simulink model "hearing_aid_final_model"  (R2018b)
settings: Solver=VariableStepAuto  StartTime=0.0  StopTime=67  RelTol=1e-3
libraries: dspvision x2, simulink x1, dspsnks4 x1, dspadpt3 x1
settings Model: Creator=User  LastModifiedBy=User

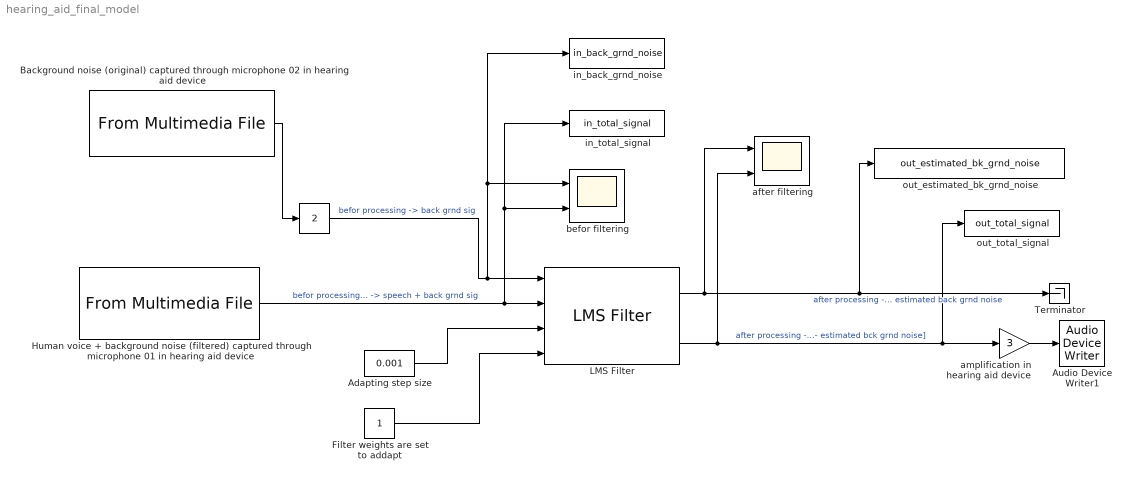
== system hearing_aid_final_model ==
  " " : simulink/Math Operations/Slider Gain  gain=2  low=0  high=5
  Adapting step size : Constant  Value=0.001  OutDataTypeStr=Inherit: Inherit via back propagation
  Audio Device Writer1 : dspsnks4/Audio Device Writer  Driver=DirectSound  Device=Default  InheritSampleRate=on  SampleRate=44100  BitDepth=16-bit integer  BufferSize=4096  NumBuffers=10  DefaultOutputChannelMapping=on  OutputChannelMapping=1:2  OutputNumUnderrunSamples=off  DriverIdx=1  DeviceWarnFlag=''
  "Background noise (original) captured through microphone 02 in hearing aid device " : dspvision/From Multimedia File  inputFilename=C:\Users\User\Documents\1.0 - Academic_Term\3 - third semester\2 - engineering system designing\000 hearing research\simulink\coffeeeshopnoise.m4a  loop=on  numPlays=inf  outputStreams=Audio only  videoDataType=single  audioDataType=double  inheritSampleTime=on  userDefinedSampleTime=1/30  noAudioOutput=off  isIntensityVideo=off  fourcc=RGB  colorVideoFormat=Separate color signals  outputEOF=off  dataOrg=Column-major  audioFrameSize=1024  computeAudioFrameSize=off  outSamplingMode=Sample based
      settings: SourceProductBaseCode=VP
  "Filter weights are set to addapt " : Constant
  Human voice + background noise (filtered) captured through microphone 01 in hearing aid device : dspvision/From Multimedia File  inputFilename=C:\Users\User\Documents\1.0 - Academic_Term\3 - third semester\2 - engineering system designing\000 hearing research\simulink\narration_plus_coffeeshop.wav  loop=on  numPlays=inf  outputStreams=Audio only  videoDataType=single  audioDataType=double  inheritSampleTime=on  userDefinedSampleTime=1/30  noAudioOutput=off  isIntensityVideo=off  fourcc=RGB  colorVideoFormat=Separate color signals  outputEOF=off  dataOrg=Column-major  audioFrameSize=1024  computeAudioFrameSize=off  outSamplingMode=Sample based
      settings: SourceProductBaseCode=VP
  LMS Filter : dspadpt3/LMS Filter  Algo=Normalized LMS  L=100  stepflag=Input port  mu=0.1  leakage=1.0  ic=0  Adapt=on  resetflag=None  weights=off  secondCoeffMode=User-defined  secondCoeffWordLength=2  secondCoeffFracLength=15  accum2Mode=User-defined  accum2FracLength=20  prodOutput2Mode=User-defined  prodOutput2FracLength=20  prodOutput3Mode=User-defined  prodOutput3FracLength=20  prodOutput4Mode=User-defined  prodOutput4FracLength=20  quotientMode=User-defined  quotientFracLength=20  roundingMode=Floor  overflowMode=off  addnparflag=off
      settings: SourceProductName=DSP System Toolbox  SourceProductBaseCode=DS
  Terminator : Terminator
  "after filtering " : Scope  NumInputPorts=2
  amplification in hearing aid device : Gain  Gain=3
  "befor filtering " : Scope  NumInputPorts=2
  "in_back_grnd_noise " : ToWorkspace  VariableName=in_back_grnd_noise  SampleTime=-1
  "in_total_signal " : ToWorkspace  VariableName=in_total_signal  SampleTime=-1
  "out_estimated_bk_grnd_noise " : ToWorkspace  VariableName=out_estimated_bk_grnd_noise  SampleTime=-1
  "out_total_signal " : ToWorkspace  VariableName=out_total_signal  SampleTime=-1
  wires:
  Human voice + background noise (filtered) captured through microphone 01 in hearing aid device/1 -> "in_total_signal "/1, "befor filtering "/2, LMS Filter/2  "befor processing -> speech + back grnd sig"
  LMS Filter/1 -> "after filtering "/1, Terminator/1, "out_estimated_bk_grnd_noise "/1  "after processing -> estimated back grnd noise"
  "Background noise (original) captured through microphone 02 in hearing aid device "/1 -> " "/1
  " "/1 -> "in_back_grnd_noise "/1, "befor filtering "/1, LMS Filter/1  "befor processing -> back grnd sig"
  LMS Filter/2 -> "after filtering "/2, amplification in hearing aid device/1, "out_total_signal "/1  "after processing -> [(speech + back grnd sig) - estimated bck grnd noise]"
  "Filter weights are set to addapt "/1 -> LMS Filter/4
  Adapting step size/1 -> LMS Filter/3
  amplification in hearing aid device/1 -> Audio Device Writer1/1
